simulink model "ZVFNEU"  (Simulink 4.00)
settings: Solver=FixedStepDiscrete  StartTime=min(t)  StopTime=max(t)  FixedStep=dt  RelTol=1e-3
values from neighbouring files (symbols this model uses):
  AB1 = zeros(r+1,1)    [ableitung_durch_zvf.m]
  AB2 = zeros(n,1)    [ableitung_durch_zvf.m]
  AD = AD+F    [zvf_design.m]
  BD = BD*K    [zvf_design.m]
  dt = 0.01    [ableitung_durch_zvf.m]
  n = 2    [ableitung_durch_zvf.m]
  r = 3    [ableitung_durch_zvf.m]
settings Model: Creator=zf1ms44  LoadExternalInput=on  ExternalInput=[t(:), u(:)]  SaveFinalState=on  LimitDataPoints=off  MaxDataPoints=size(t,1)  ExtModeAutoUpdateStatusClock=off

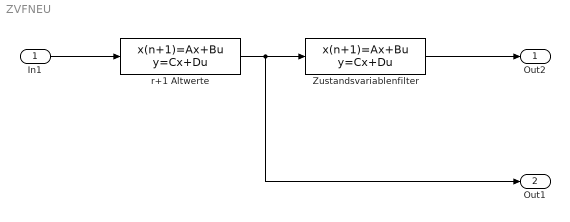
== system ZVFNEU ==
  In1 : Inport  Port=1  LatchInput=off
  Zustandsvariablenfilter : DiscreteStateSpace  A=AD  B=BD  C=eye(n)  D=zeros(n,r+1)  X0=AB2  SampleTime=dt  Realization=auto
      settings: RTWStateStorageClass=Auto
  r+1 Altwerte : DiscreteStateSpace  A=[zeros(1,r+1);[eye(r) zeros(r,1)]]  B=[1;zeros(r,1)]  C=eye(r+1)  D=zeros(r+1,1)  X0=AB1  SampleTime=dt  Realization=auto
      settings: RTWStateStorageClass=Auto
  Out2 : Outport  Port=1
  Out1 : Outport  Port=2
  wires:
  In1/1 -> r+1 Altwerte/1
  r+1 Altwerte/1 -> Out1/1, Zustandsvariablenfilter/1
  Zustandsvariablenfilter/1 -> Out2/1
